simulink model "modeloSatDead"  (R2024b)
settings: Solver=VariableStepAuto  StartTime=0.0  StopTime=10.0  RelTol=1e-3
settings Model: Creator=estel  LastModifiedBy=estel

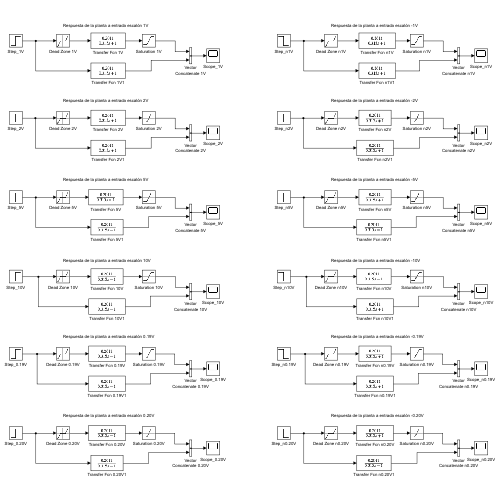
[thumbnail: Simulink's stored preview of the top-level diagram]
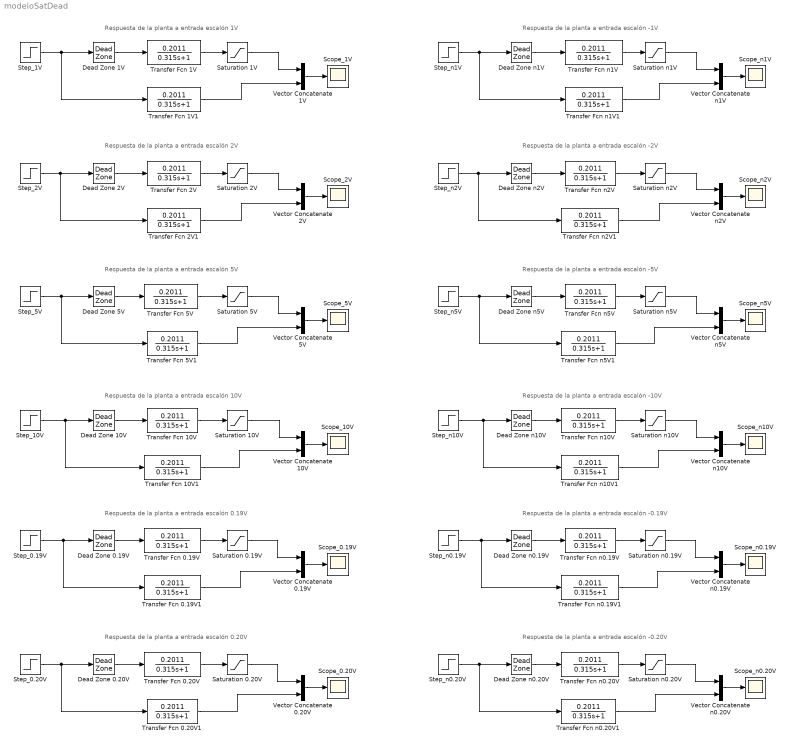
== system modeloSatDead ==
  note: Respuesta de la planta a entrada escalón 1V
  note: Respuesta de la planta a entrada escalón 2V
  note: Respuesta de la planta a entrada escalón 5V
  note: Respuesta de la planta a entrada escalón 0.20V
  note: Respuesta de la planta a entrada escalón 10V
  note: Respuesta de la planta a entrada escalón 0.19V
  note: Respuesta de la planta a entrada escalón -10V
  note: Respuesta de la planta a entrada escalón -0.19V
  note: Respuesta de la planta a entrada escalón -5V
  note: Respuesta de la planta a entrada escalón -1V
  note: Respuesta de la planta a entrada escalón -2V
  note: Respuesta de la planta a entrada escalón -0.20V
  Dead Zone 0.19V : DeadZone  LowerValue=-0.19  UpperValue=0.19
  Dead Zone 0.20V : DeadZone  LowerValue=-0.19  UpperValue=0.19
  Dead Zone 10V : DeadZone  LowerValue=-0.19  UpperValue=0.19
  Dead Zone 1V : DeadZone  LowerValue=-0.19  UpperValue=0.19
  Dead Zone 2V : DeadZone  LowerValue=-0.19  UpperValue=0.19
  Dead Zone 5V : DeadZone  LowerValue=-0.19  UpperValue=0.19
  Dead Zone n0.19V : DeadZone  LowerValue=-0.19  UpperValue=0.19
  Dead Zone n0.20V : DeadZone  LowerValue=-0.19  UpperValue=0.19
  Dead Zone n10V : DeadZone  LowerValue=-0.19  UpperValue=0.19
  Dead Zone n1V : DeadZone  LowerValue=-0.19  UpperValue=0.19
  Dead Zone n2V : DeadZone  LowerValue=-0.19  UpperValue=0.19
  Dead Zone n5V : DeadZone  LowerValue=-0.19  UpperValue=0.19
  Saturation 0.19V : Saturate  UpperLimit=10  LowerLimit=-10
  Saturation 0.20V : Saturate  UpperLimit=10  LowerLimit=-10
  Saturation 10V : Saturate  UpperLimit=10  LowerLimit=-10
  Saturation 1V : Saturate  UpperLimit=10  LowerLimit=-10
  Saturation 2V : Saturate  UpperLimit=10  LowerLimit=-10
  Saturation 5V : Saturate  UpperLimit=10  LowerLimit=-10
  Saturation n0.19V : Saturate  UpperLimit=10  LowerLimit=-10
  Saturation n0.20V : Saturate  UpperLimit=10  LowerLimit=-10
  Saturation n10V : Saturate  UpperLimit=10  LowerLimit=-10
  Saturation n1V : Saturate  UpperLimit=10  LowerLimit=-10
  Saturation n2V : Saturate  UpperLimit=10  LowerLimit=-10
  Saturation n5V : Saturate  UpperLimit=10  LowerLimit=-10
  Scope_0.19V : Scope
  Scope_0.20V : Scope
  Scope_10V : Scope
  Scope_1V : Scope
  Scope_2V : Scope
  Scope_5V : Scope
  Scope_n0.19V : Scope
  Scope_n0.20V : Scope
  Scope_n10V : Scope
  Scope_n1V : Scope
  Scope_n2V : Scope
  Scope_n5V : Scope
  Step_0.19V : Step  After=0.19  SampleTime=0
  Step_0.20V : Step  After=0.20  SampleTime=0
  Step_10V : Step  After=10  SampleTime=0
  Step_1V : Step  SampleTime=0
  Step_2V : Step  After=2  SampleTime=0
  Step_5V : Step  After=5  SampleTime=0
  Step_n0.19V : Step  After=-0.19  SampleTime=0
  Step_n0.20V : Step  After=-0.20  SampleTime=0
  Step_n10V : Step  After=-10  SampleTime=0
  Step_n1V : Step  After=-1  SampleTime=0
  Step_n2V : Step  After=-2  SampleTime=0
  Step_n5V : Step  After=-5  SampleTime=0
  Transfer Fcn 0.19V : TransferFcn  Numerator=0.2011  Denominator=[0.315 1]
  Transfer Fcn 0.19V1 : TransferFcn  Numerator=0.2011  Denominator=[0.315 1]
  Transfer Fcn 0.20V : TransferFcn  Numerator=0.2011  Denominator=[0.315 1]
  Transfer Fcn 0.20V1 : TransferFcn  Numerator=0.2011  Denominator=[0.315 1]
  Transfer Fcn 10V : TransferFcn  Numerator=0.2011  Denominator=[0.315 1]
  Transfer Fcn 10V1 : TransferFcn  Numerator=0.2011  Denominator=[0.315 1]
  Transfer Fcn 1V : TransferFcn  Numerator=0.2011  Denominator=[0.315 1]
  Transfer Fcn 1V1 : TransferFcn  Numerator=0.2011  Denominator=[0.315 1]
  Transfer Fcn 2V : TransferFcn  Numerator=0.2011  Denominator=[0.315 1]
  Transfer Fcn 2V1 : TransferFcn  Numerator=0.2011  Denominator=[0.315 1]
  Transfer Fcn 5V : TransferFcn  Numerator=0.2011  Denominator=[0.315 1]
  Transfer Fcn 5V1 : TransferFcn  Numerator=0.2011  Denominator=[0.315 1]
  Transfer Fcn n0.19V : TransferFcn  Numerator=0.2011  Denominator=[0.315 1]
  Transfer Fcn n0.19V1 : TransferFcn  Numerator=0.2011  Denominator=[0.315 1]
  Transfer Fcn n0.20V : TransferFcn  Numerator=0.2011  Denominator=[0.315 1]
  Transfer Fcn n0.20V1 : TransferFcn  Numerator=0.2011  Denominator=[0.315 1]
  Transfer Fcn n10V : TransferFcn  Numerator=0.2011  Denominator=[0.315 1]
  Transfer Fcn n10V1 : TransferFcn  Numerator=0.2011  Denominator=[0.315 1]
  Transfer Fcn n1V : TransferFcn  Numerator=0.2011  Denominator=[0.315 1]
  Transfer Fcn n1V1 : TransferFcn  Numerator=0.2011  Denominator=[0.315 1]
  Transfer Fcn n2V : TransferFcn  Numerator=0.2011  Denominator=[0.315 1]
  Transfer Fcn n2V1 : TransferFcn  Numerator=0.2011  Denominator=[0.315 1]
  Transfer Fcn n5V : TransferFcn  Numerator=0.2011  Denominator=[0.315 1]
  Transfer Fcn n5V1 : TransferFcn  Numerator=0.2011  Denominator=[0.315 1]
  Vector Concatenate 0.19V : Concatenate
  Vector Concatenate 0.20V : Concatenate
  Vector Concatenate 10V : Concatenate
  Vector Concatenate 1V : Concatenate
  Vector Concatenate 2V : Concatenate
  Vector Concatenate 5V : Concatenate
  Vector Concatenate n0.19V : Concatenate
  Vector Concatenate n0.20V : Concatenate
  Vector Concatenate n10V : Concatenate
  Vector Concatenate n1V : Concatenate
  Vector Concatenate n2V : Concatenate
  Vector Concatenate n5V : Concatenate
  wires:
  Step_1V/1 -> Dead Zone 1V/1, Transfer Fcn 1V1/1
  Transfer Fcn 1V1/1 -> Vector Concatenate 1V/2
  Vector Concatenate 1V/1 -> Scope_1V/1
  Vector Concatenate 2V/1 -> Scope_2V/1
  Transfer Fcn 2V1/1 -> Vector Concatenate 2V/2
  Step_2V/1 -> Transfer Fcn 2V1/1, Dead Zone 2V/1
  Step_5V/1 -> Dead Zone 5V/1, Transfer Fcn 5V1/1
  Transfer Fcn 5V1/1 -> Vector Concatenate 5V/2
  Vector Concatenate 5V/1 -> Scope_5V/1
  Transfer Fcn 10V1/1 -> Vector Concatenate 10V/2
  Transfer Fcn 0.20V1/1 -> Vector Concatenate 0.20V/2
  Step_0.20V/1 -> Dead Zone 0.20V/1, Transfer Fcn 0.20V1/1
  Vector Concatenate 0.20V/1 -> Scope_0.20V/1
  Step_0.19V/1 -> Dead Zone 0.19V/1, Transfer Fcn 0.19V1/1
  Transfer Fcn 0.19V1/1 -> Vector Concatenate 0.19V/2
  Vector Concatenate 10V/1 -> Scope_10V/1
  Step_10V/1 -> Dead Zone 10V/1, Transfer Fcn 10V1/1
  Vector Concatenate 0.19V/1 -> Scope_0.19V/1
  Dead Zone 0.20V/1 -> Transfer Fcn 0.20V/1
  Transfer Fcn 0.20V/1 -> Saturation 0.20V/1
  Saturation 0.20V/1 -> Vector Concatenate 0.20V/1
  Saturation 0.19V/1 -> Vector Concatenate 0.19V/1
  Transfer Fcn 0.19V/1 -> Saturation 0.19V/1
  Dead Zone 0.19V/1 -> Transfer Fcn 0.19V/1
  Saturation 10V/1 -> Vector Concatenate 10V/1
  Dead Zone 10V/1 -> Transfer Fcn 10V/1
  Transfer Fcn 10V/1 -> Saturation 10V/1
  Saturation 5V/1 -> Vector Concatenate 5V/1
  Transfer Fcn 5V/1 -> Saturation 5V/1
  Dead Zone 5V/1 -> Transfer Fcn 5V/1
  Transfer Fcn 2V/1 -> Saturation 2V/1
  Saturation 2V/1 -> Vector Concatenate 2V/1
  Dead Zone 2V/1 -> Transfer Fcn 2V/1
  Transfer Fcn 1V/1 -> Saturation 1V/1
  Saturation 1V/1 -> Vector Concatenate 1V/1
  Dead Zone 1V/1 -> Transfer Fcn 1V/1
  Dead Zone n2V/1 -> Transfer Fcn n2V/1
  Dead Zone n0.19V/1 -> Transfer Fcn n0.19V/1
  Saturation n0.19V/1 -> Vector Concatenate n0.19V/1
  Transfer Fcn n1V/1 -> Saturation n1V/1
  Transfer Fcn n5V/1 -> Saturation n5V/1
  Saturation n1V/1 -> Vector Concatenate n1V/1
  Transfer Fcn n0.20V/1 -> Saturation n0.20V/1
  Transfer Fcn n10V/1 -> Saturation n10V/1
  Dead Zone n0.20V/1 -> Transfer Fcn n0.20V/1
  Vector Concatenate n0.19V/1 -> Scope_n0.19V/1
  Dead Zone n5V/1 -> Transfer Fcn n5V/1
  Step_n10V/1 -> Dead Zone n10V/1, Transfer Fcn n10V1/1
  Vector Concatenate n10V/1 -> Scope_n10V/1
  Transfer Fcn n0.20V1/1 -> Vector Concatenate n0.20V/2
  Saturation n5V/1 -> Vector Concatenate n5V/1
  Vector Concatenate n0.20V/1 -> Scope_n0.20V/1
  Transfer Fcn n0.19V1/1 -> Vector Concatenate n0.19V/2
  Step_n0.19V/1 -> Dead Zone n0.19V/1, Transfer Fcn n0.19V1/1
  Transfer Fcn n10V1/1 -> Vector Concatenate n10V/2
  Transfer Fcn n1V1/1 -> Vector Concatenate n1V/2
  Vector Concatenate n1V/1 -> Scope_n1V/1
  Transfer Fcn n5V1/1 -> Vector Concatenate n5V/2
  Step_n5V/1 -> Dead Zone n5V/1, Transfer Fcn n5V1/1
  Step_n0.20V/1 -> Dead Zone n0.20V/1, Transfer Fcn n0.20V1/1
  Vector Concatenate n5V/1 -> Scope_n5V/1
  Saturation n0.20V/1 -> Vector Concatenate n0.20V/1
  Step_n2V/1 -> Transfer Fcn n2V1/1, Dead Zone n2V/1
  Vector Concatenate n2V/1 -> Scope_n2V/1
  Dead Zone n10V/1 -> Transfer Fcn n10V/1
  Saturation n10V/1 -> Vector Concatenate n10V/1
  Transfer Fcn n0.19V/1 -> Saturation n0.19V/1
  Saturation n2V/1 -> Vector Concatenate n2V/1
  Step_n1V/1 -> Dead Zone n1V/1, Transfer Fcn n1V1/1
  Transfer Fcn n2V/1 -> Saturation n2V/1
  Dead Zone n1V/1 -> Transfer Fcn n1V/1
  Transfer Fcn n2V1/1 -> Vector Concatenate n2V/2
